simulink model "main2_2023b"  (R2023b)
settings: Solver=ode15s  StartTime=0.0  StopTime=15  MaxStep=1e-4  RelTol=1e-3
InitFcn:
  | parametros
values from neighbouring files (symbols this model uses):
  alpha_cu = 3.9 *10^-3    (= 0.0039)    [parametros.m]
  b_l = 0.1    [parametros.m]
  b_m = 1.5 * 10^-5    (= 1.5e-05)    [parametros.m]
  C_ts = 0.818    [parametros.m]
  J_l = (m*l_cm^2 + J_cm) + (m_l * l_l^2)    (= 0.0833)    [parametros.m]
  J_m = 1.4 * 10^-5    (= 1.4e-05)    [parametros.m]
  K_e_omega = 3*3200^2    (= 30720000)    [parametros.m]
  K_e_theta = 9600    [parametros.m]
  k_l = m * g * l_cm + m_l * g * l_l    (= 2.4516625)    [parametros.m]
  L_d = 6.6 * 10^-3    (= 0.0066)    [parametros.m]
  L_ls = 0.8 * 10^-3    (= 0.0008)    [parametros.m]
  L_q = 5.8 * 10^-3    (= 0.0058)    [parametros.m]
  lambda_m = 0.016    [parametros.m]
  P_p = 3    [parametros.m]
  r = 120    [parametros.m]
  R_s_40 = 1.02    [parametros.m]
  R_ts_amb = 146.7    [parametros.m]
  Temp_s_ref = 40    [parametros.m]
libraries: simulink x6
(part 2 of 2)

== system main2_2023b/5.2.1 ids = 3/Sensores ==
  theta_m : Inport
  T_s : Inport  Port=2
  i_as : Inport  Port=3
  i_bs : Inport  Port=4
  i_cs : Inport  Port=5
  Gain{,1..4} (5 alike) : Gain
  theta_m_medida : Outport
  T_s_medida : Outport  Port=2
  i_as_medida : Outport  Port=3
  i_bs_medida : Outport  Port=4
  i_cs_medida : Outport  Port=5
  wires:
  theta_m/1 -> Gain/1
  T_s/1 -> Gain1/1
  i_as/1 -> Gain2/1
  Gain/1 -> theta_m_medida/1
  Gain1/1 -> T_s_medida/1
  Gain2/1 -> i_as_medida/1
  Gain3/1 -> i_bs_medida/1
  i_bs/1 -> Gain3/1
  i_cs/1 -> Gain4/1
  Gain4/1 -> i_cs_medida/1

== system main2_2023b/5.2.1 ids = 3/Setpoint ==
  q1* : Inport
  Derivative : Derivative
  Gain : Gain  Gain=r
  theta_m* : Outport
  omega_m* : Outport  Port=2
  wires:
  q1*/1 -> Gain/1
  Gain/1 -> Derivative/1, theta_m*/1
  Derivative/1 -> omega_m*/1

== system main2_2023b/5.2.1 ids = 3/Subsistema físico no lineal  ==
  T_l : Inport
  v_as : Inport  Port=2
  v_bs : Inport  Port=3
  v_cs : Inport  Port=4
  theta_r : Inport  Port=5
  Tº_amb : Inport  Port=6
  Subsistema electromagnético : Subsystem
  Subsistema mecánico completo : Subsystem
  Subsistema térmico : Subsystem
  TD_PARK : MATLAB Function  TreatAsAtomicUnit=on
  TI_PARK : MATLAB Function  TreatAsAtomicUnit=on
  theta_m : Outport
  T_s : Outport  Port=2
  i_as : Outport  Port=3
  i_bs : Outport  Port=4
  i_cs : Outport  Port=5
  omega_m : Outport  Port=6
  T_m : Outport  Port=7
  wires:
  theta_r/1 -> TI_PARK/4(theta_r), TD_PARK/4(theta_r)
  TI_PARK/2(fbs) -> i_bs/1
  v_cs/1 -> TD_PARK/3(fcs)
  v_as/1 -> TD_PARK/1(fas)
  TI_PARK/3(fcs) -> i_cs/1
  v_bs/1 -> TD_PARK/2(fbs)
  TI_PARK/1(fas) -> i_as/1
  TD_PARK/1(fqs) -> Subsistema electromagnético/1(v_qs^r)
  TD_PARK/2(fds) -> Subsistema electromagnético/2(v_ds^r)
  TD_PARK/3(f0s) -> Subsistema electromagnético/3(v_0s^r)
  Subsistema mecánico completo/2(omega_m(t)) -> Subsistema electromagnético/4(omega_m), omega_m/1
  Subsistema térmico/2(r_s) -> Subsistema electromagnético/5(r_s)
  Subsistema electromagnético/2(i_ds^r) -> Subsistema térmico/2(i_ds^r), TI_PARK/2(fds)
  Subsistema electromagnético/3(i_qs^r) -> Subsistema térmico/1(i_qs^r), TI_PARK/1(fqs)
  Subsistema electromagnético/1(i_0s^r) -> Subsistema térmico/3(i_0s^r), TI_PARK/3(f0s)
  Subsistema electromagnético/4(T_m) -> Subsistema mecánico completo/1(T_m), T_m/1
  T_l/1 -> Subsistema mecánico completo/2(T_l)
  Tº_amb/1 -> Subsistema térmico/4(Tº_amb)
  Subsistema térmico/1(T_s) -> T_s/1
  Subsistema mecánico completo/1(theta_m(t)) -> theta_m/1

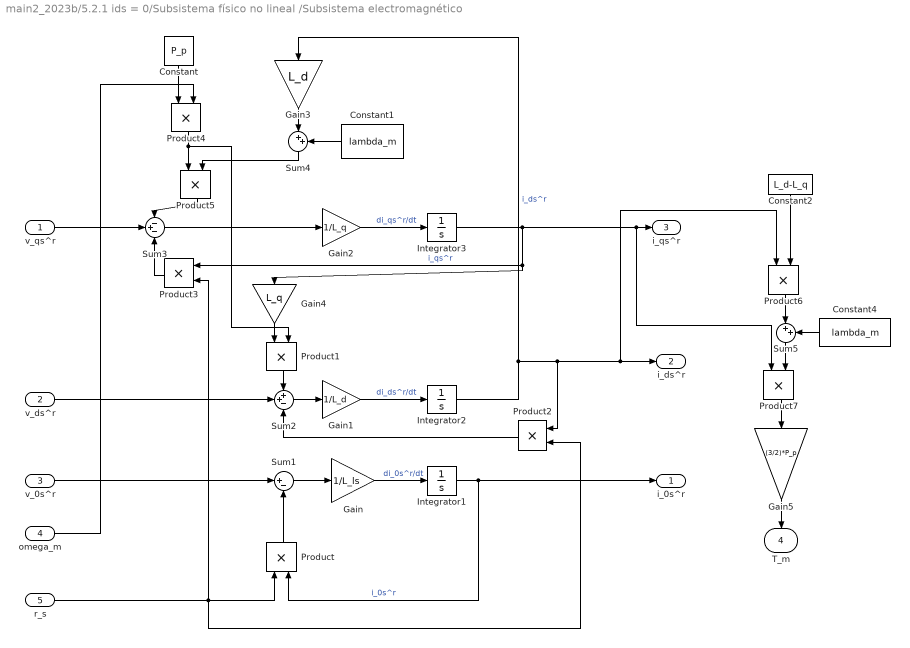
== system main2_2023b/5.2.1 ids = 0/Subsistema físico no lineal /Subsistema electromagnético ==
  v_qs^r : Inport
  v_ds^r : Inport  Port=2
  v_0s^r : Inport  Port=3
  omega_m : Inport  Port=4
  r_s : Inport  Port=5
  Constant : Constant  Value=P_p
  Constant1 : Constant  Value=lambda_m
  Constant2 : Constant  Value=L_d-L_q
  Constant4 : Constant  Value=lambda_m
  Gain : Gain  Gain=1/L_ls
  Gain1 : Gain  Gain=1/L_d
  Gain2 : Gain  Gain=1/L_q
  Gain3 : Gain  Gain=L_d
  Gain4 : Gain  Gain=L_q
  Gain5 : Gain  Gain=(3/2)*P_p
  Integrator1 : Integrator
  Integrator2 : Integrator
  Integrator3 : Integrator
  Product{,1..7} (8 alike) : Product
  Sum1 : Sum  Inputs=|+-
  Sum2 : Sum  Inputs=++-
  Sum3 : Sum  Inputs=-+-
  Sum4 : Sum  Inputs=|++
  Sum5 : Sum  Inputs=|++
  i_0s^r : Outport
  i_ds^r : Outport  Port=2
  i_qs^r : Outport  Port=3
  T_m : Outport  Port=4
  wires:
  Constant2/1 -> Product6/2
  Gain5/1 -> T_m/1
  Product5/1 -> Sum3/1
  Product2/1 -> Sum2/3
  Product6/1 -> Sum5/1
  Product1/1 -> Sum2/1
  Gain4/1 -> Product1/1
  Constant4/1 -> Sum5/2
  Sum3/1 -> Gain2/1
  Constant1/1 -> Sum4/2
  Integrator1/1 -> i_0s^r/1, Product/2  "i_0s^r"
  v_ds^r/1 -> Sum2/2
  Product4/1 -> Product1/2, Product5/1
  Sum5/1 -> Product7/2
  Product7/1 -> Gain5/1
  Integrator2/1 -> Gain3/1, Product2/1, Product6/1, i_ds^r/1  "i_ds^r"
  Sum4/1 -> Product5/2
  Product/1 -> Sum1/2
  Integrator3/1 -> Product3/1, Gain4/1, Product7/1, i_qs^r/1  "i_qs^r"
  Product3/1 -> Sum3/3
  Gain/1 -> Integrator1/1  "di_0s^r/dt"
  Gain3/1 -> Sum4/1
  omega_m/1 -> Product4/2
  Constant/1 -> Product4/1
  Sum1/1 -> Gain/1
  r_s/1 -> Product3/2, Product2/2, Product/1
  v_qs^r/1 -> Sum3/2
  Gain2/1 -> Integrator3/1  "di_qs^r/dt"
  v_0s^r/1 -> Sum1/1
  Gain1/1 -> Integrator2/1  "di_ds^r/dt"
  Sum2/1 -> Gain1/1

== system main2_2023b/5.2.1 ids = 0/Subsistema físico no lineal /Subsistema mecánico completo ==
  T_m : Inport
  T_l : Inport  Port=2
  Gain : Gain  Gain=b_m +( b_l / (r^2))
  Gain1 : Gain  Gain=1/r
  Gain2 : Gain  Gain=1/(J_m + J_l / (r^2))
  Sum : Sum  Inputs=-+-
  omega_m(0) = 0 : Integrator
  theta_m(0) = 0 : Integrator
  theta_m(t) : Outport
  omega_m(t) : Outport  Port=2
  wires:
  Gain2/1 -> omega_m(0) = 0/1  "domega_m(t)/dt"
  Gain1/1 -> Sum/1
  theta_m(0) = 0/1 -> theta_m(t)/1  "theta_m(t)"
  omega_m(0) = 0/1 -> omega_m(t)/1, Gain/1, theta_m(0) = 0/1  "omega_m(t)"
  Sum/1 -> Gain2/1
  Gain/1 -> Sum/3
  T_l/1 -> Gain1/1
  T_m/1 -> Sum/2

== system main2_2023b/5.2.1 ids = 0/Subsistema físico no lineal /Subsistema térmico ==
  i_qs^r : Inport
  i_ds^r : Inport  Port=2
  i_0s^r : Inport  Port=3
  Tº_amb : Inport  Port=4
  CI = 40ºC : Integrator  InitialCondition=40
  Constant : Constant
  Gain : Gain  Gain=1/C_ts
  Gain1 : Gain  Gain=2
  Gain2 : Gain  Gain=3/2
  Gain3 : Gain  Gain=1/R_ts_amb
  Gain4 : Gain  Gain=alpha_cu
  Gain5 : Gain  Gain=R_s_40
  Product : Product
  Square : Math  Operator=square
  Square1 : Math  Operator=square
  Square2 : Math  Operator=square
  Sum : Sum  Inputs=+++
  Sum1 : Sum  Inputs=|+-
  Sum2 : Sum  Inputs=|-+
  Sum3 : Sum  Inputs=|++
  T_s : Outport
  r_s : Outport  Port=2
  wires:
  CI = 40ºC/1 -> Sum2/2, T_s/1
  Gain/1 -> CI = 40ºC/1
  Sum1/1 -> Gain/1
  i_qs^r/1 -> Square/1
  i_ds^r/1 -> Square1/1
  i_0s^r/1 -> Square2/1
  Square2/1 -> Gain1/1
  Square/1 -> Sum/1
  Square1/1 -> Sum/2
  Gain1/1 -> Sum/3
  Gain5/1 -> r_s/1, Gain2/1
  Gain2/1 -> Product/2
  Sum/1 -> Product/1
  Product/1 -> Sum1/1
  Tº_amb/1 -> Sum2/1
  Sum2/1 -> Gain4/1, Gain3/1
  Gain3/1 -> Sum1/2
  Gain4/1 -> Sum3/1
  Constant/1 -> Sum3/2
  Sum3/1 -> Gain5/1

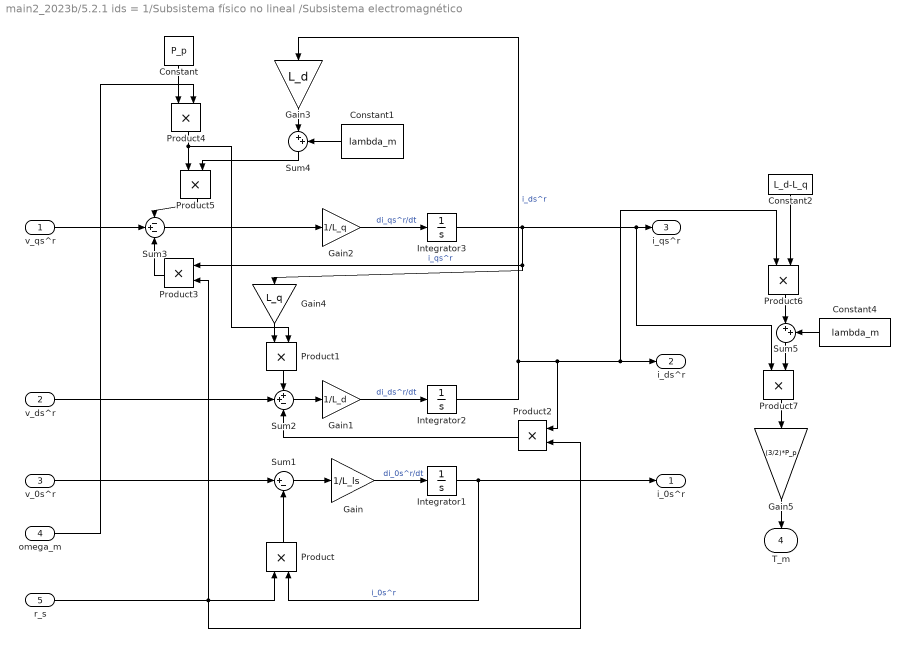
== system main2_2023b/5.2.1 ids = 1/Subsistema físico no lineal /Subsistema electromagnético ==
  v_qs^r : Inport
  v_ds^r : Inport  Port=2
  v_0s^r : Inport  Port=3
  omega_m : Inport  Port=4
  r_s : Inport  Port=5
  Constant : Constant  Value=P_p
  Constant1 : Constant  Value=lambda_m
  Constant2 : Constant  Value=L_d-L_q
  Constant4 : Constant  Value=lambda_m
  Gain : Gain  Gain=1/L_ls
  Gain1 : Gain  Gain=1/L_d
  Gain2 : Gain  Gain=1/L_q
  Gain3 : Gain  Gain=L_d
  Gain4 : Gain  Gain=L_q
  Gain5 : Gain  Gain=(3/2)*P_p
  Integrator1 : Integrator
  Integrator2 : Integrator
  Integrator3 : Integrator
  Product{,1..7} (8 alike) : Product
  Sum1 : Sum  Inputs=|+-
  Sum2 : Sum  Inputs=++-
  Sum3 : Sum  Inputs=-+-
  Sum4 : Sum  Inputs=|++
  Sum5 : Sum  Inputs=|++
  i_0s^r : Outport
  i_ds^r : Outport  Port=2
  i_qs^r : Outport  Port=3
  T_m : Outport  Port=4
  wires:
  Constant2/1 -> Product6/2
  Gain5/1 -> T_m/1
  Product5/1 -> Sum3/1
  Product2/1 -> Sum2/3
  Product6/1 -> Sum5/1
  Product1/1 -> Sum2/1
  Gain4/1 -> Product1/1
  Constant4/1 -> Sum5/2
  Sum3/1 -> Gain2/1
  Constant1/1 -> Sum4/2
  Integrator1/1 -> i_0s^r/1, Product/2  "i_0s^r"
  v_ds^r/1 -> Sum2/2
  Product4/1 -> Product1/2, Product5/1
  Sum5/1 -> Product7/2
  Product7/1 -> Gain5/1
  Integrator2/1 -> Gain3/1, Product2/1, Product6/1, i_ds^r/1  "i_ds^r"
  Sum4/1 -> Product5/2
  Product/1 -> Sum1/2
  Integrator3/1 -> Product3/1, Gain4/1, Product7/1, i_qs^r/1  "i_qs^r"
  Product3/1 -> Sum3/3
  Gain/1 -> Integrator1/1  "di_0s^r/dt"
  Gain3/1 -> Sum4/1
  omega_m/1 -> Product4/2
  Constant/1 -> Product4/1
  Sum1/1 -> Gain/1
  r_s/1 -> Product3/2, Product2/2, Product/1
  v_qs^r/1 -> Sum3/2
  Gain2/1 -> Integrator3/1  "di_qs^r/dt"
  v_0s^r/1 -> Sum1/1
  Gain1/1 -> Integrator2/1  "di_ds^r/dt"
  Sum2/1 -> Gain1/1

== system main2_2023b/5.2.1 ids = 1/Subsistema físico no lineal /Subsistema mecánico completo ==
  T_m : Inport
  T_l : Inport  Port=2
  Gain : Gain  Gain=b_m +( b_l / (r^2))
  Gain1 : Gain  Gain=1/r
  Gain2 : Gain  Gain=1/(J_m + J_l / (r^2))
  Sum : Sum  Inputs=-+-
  omega_m(0) = 0 : Integrator
  theta_m(0) = 0 : Integrator
  theta_m(t) : Outport
  omega_m(t) : Outport  Port=2
  wires:
  Gain2/1 -> omega_m(0) = 0/1  "domega_m(t)/dt"
  Gain1/1 -> Sum/1
  theta_m(0) = 0/1 -> theta_m(t)/1  "theta_m(t)"
  omega_m(0) = 0/1 -> omega_m(t)/1, Gain/1, theta_m(0) = 0/1  "omega_m(t)"
  Sum/1 -> Gain2/1
  Gain/1 -> Sum/3
  T_l/1 -> Gain1/1
  T_m/1 -> Sum/2

== system main2_2023b/5.2.1 ids = 1/Subsistema físico no lineal /Subsistema térmico ==
  i_qs^r : Inport
  i_ds^r : Inport  Port=2
  i_0s^r : Inport  Port=3
  Tº_amb : Inport  Port=4
  CI = 40ºC : Integrator  InitialCondition=40
  Constant : Constant
  Gain : Gain  Gain=1/C_ts
  Gain1 : Gain  Gain=2
  Gain2 : Gain  Gain=3/2
  Gain3 : Gain  Gain=1/R_ts_amb
  Gain4 : Gain  Gain=alpha_cu
  Gain5 : Gain  Gain=R_s_40
  Product : Product
  Square : Math  Operator=square
  Square1 : Math  Operator=square
  Square2 : Math  Operator=square
  Sum : Sum  Inputs=+++
  Sum1 : Sum  Inputs=|+-
  Sum2 : Sum  Inputs=|-+
  Sum3 : Sum  Inputs=|++
  T_s : Outport
  r_s : Outport  Port=2
  wires:
  CI = 40ºC/1 -> Sum2/2, T_s/1
  Gain/1 -> CI = 40ºC/1
  Sum1/1 -> Gain/1
  i_qs^r/1 -> Square/1
  i_ds^r/1 -> Square1/1
  i_0s^r/1 -> Square2/1
  Square2/1 -> Gain1/1
  Square/1 -> Sum/1
  Square1/1 -> Sum/2
  Gain1/1 -> Sum/3
  Gain5/1 -> r_s/1, Gain2/1
  Gain2/1 -> Product/2
  Sum/1 -> Product/1
  Product/1 -> Sum1/1
  Tº_amb/1 -> Sum2/1
  Sum2/1 -> Gain4/1, Gain3/1
  Gain3/1 -> Sum1/2
  Gain4/1 -> Sum3/1
  Constant/1 -> Sum3/2
  Sum3/1 -> Gain5/1

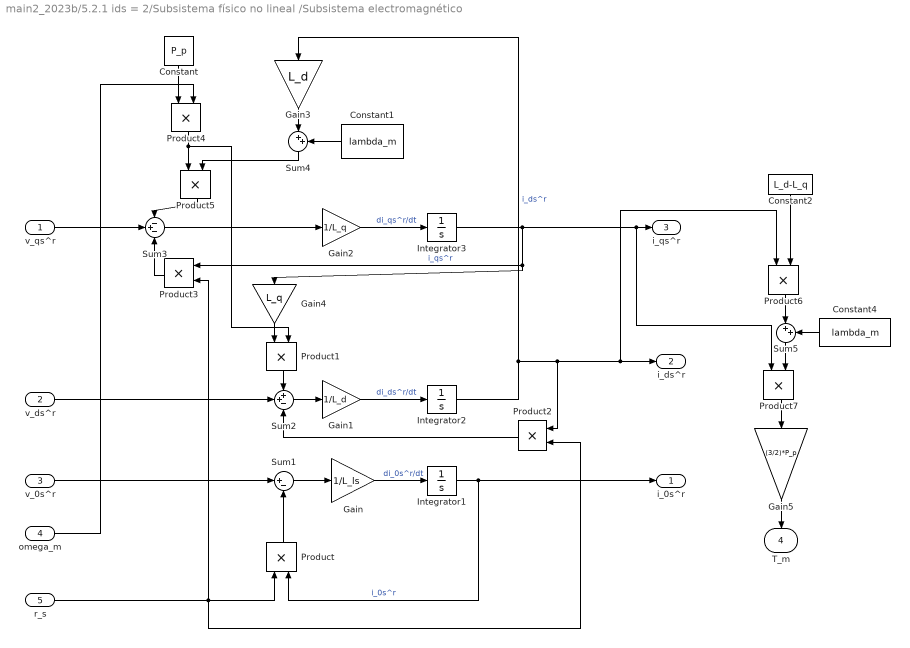
== system main2_2023b/5.2.1 ids = 2/Subsistema físico no lineal /Subsistema electromagnético ==
  v_qs^r : Inport
  v_ds^r : Inport  Port=2
  v_0s^r : Inport  Port=3
  omega_m : Inport  Port=4
  r_s : Inport  Port=5
  Constant : Constant  Value=P_p
  Constant1 : Constant  Value=lambda_m
  Constant2 : Constant  Value=L_d-L_q
  Constant4 : Constant  Value=lambda_m
  Gain : Gain  Gain=1/L_ls
  Gain1 : Gain  Gain=1/L_d
  Gain2 : Gain  Gain=1/L_q
  Gain3 : Gain  Gain=L_d
  Gain4 : Gain  Gain=L_q
  Gain5 : Gain  Gain=(3/2)*P_p
  Integrator1 : Integrator
  Integrator2 : Integrator
  Integrator3 : Integrator
  Product{,1..7} (8 alike) : Product
  Sum1 : Sum  Inputs=|+-
  Sum2 : Sum  Inputs=++-
  Sum3 : Sum  Inputs=-+-
  Sum4 : Sum  Inputs=|++
  Sum5 : Sum  Inputs=|++
  i_0s^r : Outport
  i_ds^r : Outport  Port=2
  i_qs^r : Outport  Port=3
  T_m : Outport  Port=4
  wires:
  Constant2/1 -> Product6/2
  Gain5/1 -> T_m/1
  Product5/1 -> Sum3/1
  Product2/1 -> Sum2/3
  Product6/1 -> Sum5/1
  Product1/1 -> Sum2/1
  Gain4/1 -> Product1/1
  Constant4/1 -> Sum5/2
  Sum3/1 -> Gain2/1
  Constant1/1 -> Sum4/2
  Integrator1/1 -> i_0s^r/1, Product/2  "i_0s^r"
  v_ds^r/1 -> Sum2/2
  Product4/1 -> Product1/2, Product5/1
  Sum5/1 -> Product7/2
  Product7/1 -> Gain5/1
  Integrator2/1 -> Gain3/1, Product2/1, Product6/1, i_ds^r/1  "i_ds^r"
  Sum4/1 -> Product5/2
  Product/1 -> Sum1/2
  Integrator3/1 -> Product3/1, Gain4/1, Product7/1, i_qs^r/1  "i_qs^r"
  Product3/1 -> Sum3/3
  Gain/1 -> Integrator1/1  "di_0s^r/dt"
  Gain3/1 -> Sum4/1
  omega_m/1 -> Product4/2
  Constant/1 -> Product4/1
  Sum1/1 -> Gain/1
  r_s/1 -> Product3/2, Product2/2, Product/1
  v_qs^r/1 -> Sum3/2
  Gain2/1 -> Integrator3/1  "di_qs^r/dt"
  v_0s^r/1 -> Sum1/1
  Gain1/1 -> Integrator2/1  "di_ds^r/dt"
  Sum2/1 -> Gain1/1

== system main2_2023b/5.2.1 ids = 2/Subsistema físico no lineal /Subsistema mecánico completo ==
  T_m : Inport
  T_l : Inport  Port=2
  Gain : Gain  Gain=b_m +( b_l / (r^2))
  Gain1 : Gain  Gain=1/r
  Gain2 : Gain  Gain=1/(J_m + J_l / (r^2))
  Sum : Sum  Inputs=-+-
  omega_m(0) = 0 : Integrator
  theta_m(0) = 0 : Integrator
  theta_m(t) : Outport
  omega_m(t) : Outport  Port=2
  wires:
  Gain2/1 -> omega_m(0) = 0/1  "domega_m(t)/dt"
  Gain1/1 -> Sum/1
  theta_m(0) = 0/1 -> theta_m(t)/1  "theta_m(t)"
  omega_m(0) = 0/1 -> omega_m(t)/1, Gain/1, theta_m(0) = 0/1  "omega_m(t)"
  Sum/1 -> Gain2/1
  Gain/1 -> Sum/3
  T_l/1 -> Gain1/1
  T_m/1 -> Sum/2

== system main2_2023b/5.2.1 ids = 2/Subsistema físico no lineal /Subsistema térmico ==
  i_qs^r : Inport
  i_ds^r : Inport  Port=2
  i_0s^r : Inport  Port=3
  Tº_amb : Inport  Port=4
  CI = 40ºC : Integrator  InitialCondition=40
  Constant : Constant
  Gain : Gain  Gain=1/C_ts
  Gain1 : Gain  Gain=2
  Gain2 : Gain  Gain=3/2
  Gain3 : Gain  Gain=1/R_ts_amb
  Gain4 : Gain  Gain=alpha_cu
  Gain5 : Gain  Gain=R_s_40
  Product : Product
  Square : Math  Operator=square
  Square1 : Math  Operator=square
  Square2 : Math  Operator=square
  Sum : Sum  Inputs=+++
  Sum1 : Sum  Inputs=|+-
  Sum2 : Sum  Inputs=|-+
  Sum3 : Sum  Inputs=|++
  T_s : Outport
  r_s : Outport  Port=2
  wires:
  CI = 40ºC/1 -> Sum2/2, T_s/1
  Gain/1 -> CI = 40ºC/1
  Sum1/1 -> Gain/1
  i_qs^r/1 -> Square/1
  i_ds^r/1 -> Square1/1
  i_0s^r/1 -> Square2/1
  Square2/1 -> Gain1/1
  Square/1 -> Sum/1
  Square1/1 -> Sum/2
  Gain1/1 -> Sum/3
  Gain5/1 -> r_s/1, Gain2/1
  Gain2/1 -> Product/2
  Sum/1 -> Product/1
  Product/1 -> Sum1/1
  Tº_amb/1 -> Sum2/1
  Sum2/1 -> Gain4/1, Gain3/1
  Gain3/1 -> Sum1/2
  Gain4/1 -> Sum3/1
  Constant/1 -> Sum3/2
  Sum3/1 -> Gain5/1

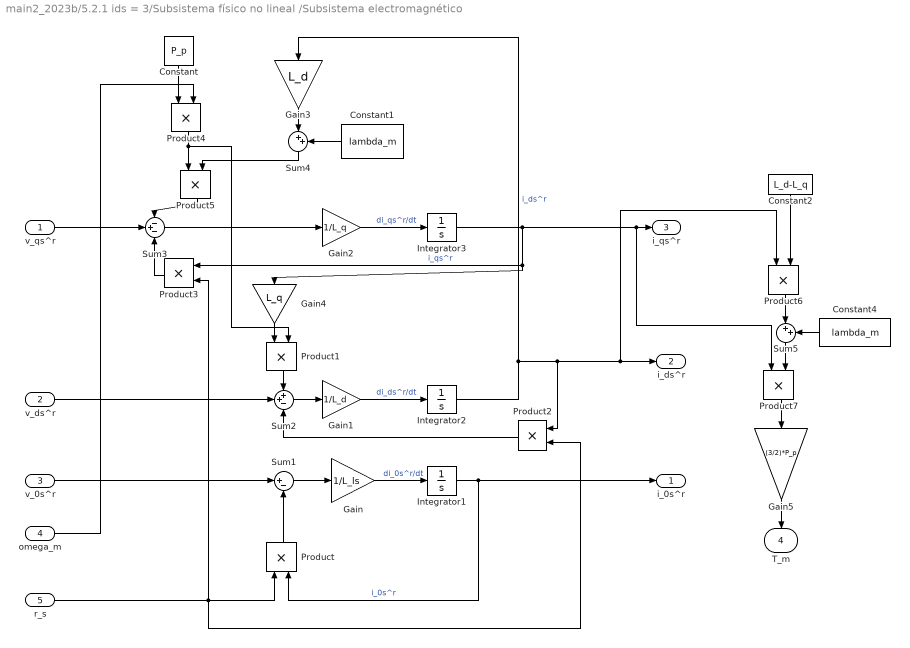
== system main2_2023b/5.2.1 ids = 3/Subsistema físico no lineal /Subsistema electromagnético ==
  v_qs^r : Inport
  v_ds^r : Inport  Port=2
  v_0s^r : Inport  Port=3
  omega_m : Inport  Port=4
  r_s : Inport  Port=5
  Constant : Constant  Value=P_p
  Constant1 : Constant  Value=lambda_m
  Constant2 : Constant  Value=L_d-L_q
  Constant4 : Constant  Value=lambda_m
  Gain : Gain  Gain=1/L_ls
  Gain1 : Gain  Gain=1/L_d
  Gain2 : Gain  Gain=1/L_q
  Gain3 : Gain  Gain=L_d
  Gain4 : Gain  Gain=L_q
  Gain5 : Gain  Gain=(3/2)*P_p
  Integrator1 : Integrator
  Integrator2 : Integrator
  Integrator3 : Integrator
  Product{,1..7} (8 alike) : Product
  Sum1 : Sum  Inputs=|+-
  Sum2 : Sum  Inputs=++-
  Sum3 : Sum  Inputs=-+-
  Sum4 : Sum  Inputs=|++
  Sum5 : Sum  Inputs=|++
  i_0s^r : Outport
  i_ds^r : Outport  Port=2
  i_qs^r : Outport  Port=3
  T_m : Outport  Port=4
  wires:
  Constant2/1 -> Product6/2
  Gain5/1 -> T_m/1
  Product5/1 -> Sum3/1
  Product2/1 -> Sum2/3
  Product6/1 -> Sum5/1
  Product1/1 -> Sum2/1
  Gain4/1 -> Product1/1
  Constant4/1 -> Sum5/2
  Sum3/1 -> Gain2/1
  Constant1/1 -> Sum4/2
  Integrator1/1 -> i_0s^r/1, Product/2  "i_0s^r"
  v_ds^r/1 -> Sum2/2
  Product4/1 -> Product1/2, Product5/1
  Sum5/1 -> Product7/2
  Product7/1 -> Gain5/1
  Integrator2/1 -> Gain3/1, Product2/1, Product6/1, i_ds^r/1  "i_ds^r"
  Sum4/1 -> Product5/2
  Product/1 -> Sum1/2
  Integrator3/1 -> Product3/1, Gain4/1, Product7/1, i_qs^r/1  "i_qs^r"
  Product3/1 -> Sum3/3
  Gain/1 -> Integrator1/1  "di_0s^r/dt"
  Gain3/1 -> Sum4/1
  omega_m/1 -> Product4/2
  Constant/1 -> Product4/1
  Sum1/1 -> Gain/1
  r_s/1 -> Product3/2, Product2/2, Product/1
  v_qs^r/1 -> Sum3/2
  Gain2/1 -> Integrator3/1  "di_qs^r/dt"
  v_0s^r/1 -> Sum1/1
  Gain1/1 -> Integrator2/1  "di_ds^r/dt"
  Sum2/1 -> Gain1/1

== system main2_2023b/5.2.1 ids = 3/Subsistema físico no lineal /Subsistema mecánico completo ==
  T_m : Inport
  T_l : Inport  Port=2
  Gain : Gain  Gain=b_m +( b_l / (r^2))
  Gain1 : Gain  Gain=1/r
  Gain2 : Gain  Gain=1/(J_m + J_l / (r^2))
  Sum : Sum  Inputs=-+-
  omega_m(0) = 0 : Integrator
  theta_m(0) = 0 : Integrator
  theta_m(t) : Outport
  omega_m(t) : Outport  Port=2
  wires:
  Gain2/1 -> omega_m(0) = 0/1  "domega_m(t)/dt"
  Gain1/1 -> Sum/1
  theta_m(0) = 0/1 -> theta_m(t)/1  "theta_m(t)"
  omega_m(0) = 0/1 -> omega_m(t)/1, Gain/1, theta_m(0) = 0/1  "omega_m(t)"
  Sum/1 -> Gain2/1
  Gain/1 -> Sum/3
  T_l/1 -> Gain1/1
  T_m/1 -> Sum/2

== system main2_2023b/5.2.1 ids = 3/Subsistema físico no lineal /Subsistema térmico ==
  i_qs^r : Inport
  i_ds^r : Inport  Port=2
  i_0s^r : Inport  Port=3
  Tº_amb : Inport  Port=4
  CI = 40ºC : Integrator  InitialCondition=40
  Constant : Constant
  Gain : Gain  Gain=1/C_ts
  Gain1 : Gain  Gain=2
  Gain2 : Gain  Gain=3/2
  Gain3 : Gain  Gain=1/R_ts_amb
  Gain4 : Gain  Gain=alpha_cu
  Gain5 : Gain  Gain=R_s_40
  Product : Product
  Square : Math  Operator=square
  Square1 : Math  Operator=square
  Square2 : Math  Operator=square
  Sum : Sum  Inputs=+++
  Sum1 : Sum  Inputs=|+-
  Sum2 : Sum  Inputs=|-+
  Sum3 : Sum  Inputs=|++
  T_s : Outport
  r_s : Outport  Port=2
  wires:
  CI = 40ºC/1 -> Sum2/2, T_s/1
  Gain/1 -> CI = 40ºC/1
  Sum1/1 -> Gain/1
  i_qs^r/1 -> Square/1
  i_ds^r/1 -> Square1/1
  i_0s^r/1 -> Square2/1
  Square2/1 -> Gain1/1
  Square/1 -> Sum/1
  Square1/1 -> Sum/2
  Gain1/1 -> Sum/3
  Gain5/1 -> r_s/1, Gain2/1
  Gain2/1 -> Product/2
  Sum/1 -> Product/1
  Product/1 -> Sum1/1
  Tº_amb/1 -> Sum2/1
  Sum2/1 -> Gain4/1, Gain3/1
  Gain3/1 -> Sum1/2
  Gain4/1 -> Sum3/1
  Constant/1 -> Sum3/2
  Sum3/1 -> Gain5/1

== matlab function main2_2023b/5.2.1 ids = 3/TD_PARK ==
  data: fas input; fqs output; fbs input; fcs input; theta_r input; fds output; f0s output
function [fqs, fds, f0s] = TD_PARK(fas, fbs, fcs, theta_r)

    fabcs = [fas; fbs; fcs];

    Ks = 2/3*[cos(theta_r) cos(theta_r - 2*pi/3) cos(theta_r + 2*pi/3)
          sin(theta_r) sin(theta_r - 2*pi/3) sin(theta_r + 2*pi/3) 
          1/2          1/2                   1/2];

    fqd0s = Ks * fabcs;

    fqs = fqd0s(1);
    fds = fqd0s(2);
    f0s = fqd0s(3);

end

== matlab function main2_2023b/5.2.1 ids = 0/Subsistema físico no lineal /TD_PARK ==
  data: fas input; fqs output; fbs input; fcs input; theta_r input; fds output; f0s output
function [fqs, fds, f0s] = TD_PARK(fas, fbs, fcs, theta_r)

    fabcs = [fas; fbs; fcs];

    Ks = 2/3*[cos(theta_r) cos(theta_r - 2*pi/3) cos(theta_r + 2*pi/3)
          sin(theta_r) sin(theta_r - 2*pi/3) sin(theta_r + 2*pi/3) 
          1/2          1/2                   1/2];

    fqd0s = Ks * fabcs;

    fqs = fqd0s(1);
    fds = fqd0s(2);
    f0s = fqd0s(3);

end

== matlab function main2_2023b/5.2.1 ids = 3/TI_PARK1 ==
  data: fqs input; fas output; fds input; f0s input; theta_r input; fbs output; fcs output
function [fas, fbs, fcs] = TI_PARK(fqs, fds, f0s , theta_r)

    fqd0s = [fqs; fds; f0s];

    Ks = [cos(theta_r)         sin(theta_r)             1
          cos(theta_r - 2*pi/3) sin(theta_r - 2*pi/3)    1
          cos(theta_r + 2*pi/3) sin(theta_r + 2*pi/3)    1];

    fabcs = Ks * fqd0s;

    fas = fabcs(1);
    fbs = fabcs(2);
    fcs = fabcs(3);

end

== matlab function main2_2023b/5.2.1 ids = 1/Subsistema físico no lineal /TD_PARK ==
  data: fas input; fqs output; fbs input; fcs input; theta_r input; fds output; f0s output
function [fqs, fds, f0s] = TD_PARK(fas, fbs, fcs, theta_r)

    fabcs = [fas; fbs; fcs];

    Ks = 2/3*[cos(theta_r) cos(theta_r - 2*pi/3) cos(theta_r + 2*pi/3)
          sin(theta_r) sin(theta_r - 2*pi/3) sin(theta_r + 2*pi/3) 
          1/2          1/2                   1/2];

    fqd0s = Ks * fabcs;

    fqs = fqd0s(1);
    fds = fqd0s(2);
    f0s = fqd0s(3);

end

== matlab function main2_2023b/5.2.1 ids = 1/Subsistema físico no lineal /TI_PARK ==
  data: fqs input; fas output; fds input; f0s input; theta_r input; fbs output; fcs output
function [fas, fbs, fcs] = TI_PARK(fqs, fds, f0s , theta_r)

    fqd0s = [fqs; fds; f0s];

    Ks = [cos(theta_r)         sin(theta_r)             1
          cos(theta_r - 2*pi/3) sin(theta_r - 2*pi/3)    1
          cos(theta_r + 2*pi/3) sin(theta_r + 2*pi/3)    1];

    fabcs = Ks * fqd0s;

    fas = fabcs(1);
    fbs = fabcs(2);
    fcs = fabcs(3);

end

== matlab function main2_2023b/5.2.1 ids = 0/TI_PARK1 ==
  data: fqs input; fas output; fds input; f0s input; theta_r input; fbs output; fcs output
function [fas, fbs, fcs] = TI_PARK(fqs, fds, f0s , theta_r)

    fqd0s = [fqs; fds; f0s];

    Ks = [cos(theta_r)         sin(theta_r)             1
          cos(theta_r - 2*pi/3) sin(theta_r - 2*pi/3)    1
          cos(theta_r + 2*pi/3) sin(theta_r + 2*pi/3)    1];

    fabcs = Ks * fqd0s;

    fas = fabcs(1);
    fbs = fabcs(2);
    fcs = fabcs(3);

end

== matlab function main2_2023b/5.2.1 ids = 0/TD_PARK ==
  data: fas input; fqs output; fbs input; fcs input; theta_r input; fds output; f0s output
function [fqs, fds, f0s] = TD_PARK(fas, fbs, fcs, theta_r)

    fabcs = [fas; fbs; fcs];

    Ks = 2/3*[cos(theta_r) cos(theta_r - 2*pi/3) cos(theta_r + 2*pi/3)
          sin(theta_r) sin(theta_r - 2*pi/3) sin(theta_r + 2*pi/3) 
          1/2          1/2                   1/2];

    fqd0s = Ks * fabcs;

    fqs = fqd0s(1);
    fds = fqd0s(2);
    f0s = fqd0s(3);

end

== matlab function main2_2023b/5.2.1 ids = 1/TD_PARK ==
  data: fas input; fqs output; fbs input; fcs input; theta_r input; fds output; f0s output
function [fqs, fds, f0s] = TD_PARK(fas, fbs, fcs, theta_r)

    fabcs = [fas; fbs; fcs];

    Ks = 2/3*[cos(theta_r) cos(theta_r - 2*pi/3) cos(theta_r + 2*pi/3)
          sin(theta_r) sin(theta_r - 2*pi/3) sin(theta_r + 2*pi/3) 
          1/2          1/2                   1/2];

    fqd0s = Ks * fabcs;

    fqs = fqd0s(1);
    fds = fqd0s(2);
    f0s = fqd0s(3);

end

== matlab function main2_2023b/5.2.1 ids = 1/TI_PARK1 ==
  data: fqs input; fas output; fds input; f0s input; theta_r input; fbs output; fcs output
function [fas, fbs, fcs] = TI_PARK(fqs, fds, f0s , theta_r)

    fqd0s = [fqs; fds; f0s];

    Ks = [cos(theta_r)         sin(theta_r)             1
          cos(theta_r - 2*pi/3) sin(theta_r - 2*pi/3)    1
          cos(theta_r + 2*pi/3) sin(theta_r + 2*pi/3)    1];

    fabcs = Ks * fqd0s;

    fas = fabcs(1);
    fbs = fabcs(2);
    fcs = fabcs(3);

end

== matlab function main2_2023b/5.2.1 ids = 0/Subsistema físico no lineal /TI_PARK ==
  data: fqs input; fas output; fds input; f0s input; theta_r input; fbs output; fcs output
function [fas, fbs, fcs] = TI_PARK(fqs, fds, f0s , theta_r)

    fqd0s = [fqs; fds; f0s];

    Ks = [cos(theta_r)         sin(theta_r)             1
          cos(theta_r - 2*pi/3) sin(theta_r - 2*pi/3)    1
          cos(theta_r + 2*pi/3) sin(theta_r + 2*pi/3)    1];

    fabcs = Ks * fqd0s;

    fas = fabcs(1);
    fbs = fabcs(2);
    fcs = fabcs(3);

end

== matlab function main2_2023b/5.2.1 ids = 2/Subsistema físico no lineal /TD_PARK ==
  data: fas input; fqs output; fbs input; fcs input; theta_r input; fds output; f0s output
function [fqs, fds, f0s] = TD_PARK(fas, fbs, fcs, theta_r)

    fabcs = [fas; fbs; fcs];

    Ks = 2/3*[cos(theta_r) cos(theta_r - 2*pi/3) cos(theta_r + 2*pi/3)
          sin(theta_r) sin(theta_r - 2*pi/3) sin(theta_r + 2*pi/3) 
          1/2          1/2                   1/2];

    fqd0s = Ks * fabcs;

    fqs = fqd0s(1);
    fds = fqd0s(2);
    f0s = fqd0s(3);

end

== matlab function main2_2023b/5.2.1 ids = 2/Subsistema físico no lineal /TI_PARK ==
  data: fqs input; fas output; fds input; f0s input; theta_r input; fbs output; fcs output
function [fas, fbs, fcs] = TI_PARK(fqs, fds, f0s , theta_r)

    fqd0s = [fqs; fds; f0s];

    Ks = [cos(theta_r)         sin(theta_r)             1
          cos(theta_r - 2*pi/3) sin(theta_r - 2*pi/3)    1
          cos(theta_r + 2*pi/3) sin(theta_r + 2*pi/3)    1];

    fabcs = Ks * fqd0s;

    fas = fabcs(1);
    fbs = fabcs(2);
    fcs = fabcs(3);

end

== matlab function main2_2023b/5.2.1 ids = 2/TD_PARK ==
  data: fas input; fqs output; fbs input; fcs input; theta_r input; fds output; f0s output
function [fqs, fds, f0s] = TD_PARK(fas, fbs, fcs, theta_r)

    fabcs = [fas; fbs; fcs];

    Ks = 2/3*[cos(theta_r) cos(theta_r - 2*pi/3) cos(theta_r + 2*pi/3)
          sin(theta_r) sin(theta_r - 2*pi/3) sin(theta_r + 2*pi/3) 
          1/2          1/2                   1/2];

    fqd0s = Ks * fabcs;

    fqs = fqd0s(1);
    fds = fqd0s(2);
    f0s = fqd0s(3);

end

== matlab function main2_2023b/5.2.1 ids = 2/TI_PARK1 ==
  data: fqs input; fas output; fds input; f0s input; theta_r input; fbs output; fcs output
function [fas, fbs, fcs] = TI_PARK(fqs, fds, f0s , theta_r)

    fqd0s = [fqs; fds; f0s];

    Ks = [cos(theta_r)         sin(theta_r)             1
          cos(theta_r - 2*pi/3) sin(theta_r - 2*pi/3)    1
          cos(theta_r + 2*pi/3) sin(theta_r + 2*pi/3)    1];

    fabcs = Ks * fqd0s;

    fas = fabcs(1);
    fbs = fabcs(2);
    fcs = fabcs(3);

end

== matlab function main2_2023b/5.2.1 ids = 3/Subsistema físico no lineal /TD_PARK ==
  data: fas input; fqs output; fbs input; fcs input; theta_r input; fds output; f0s output
function [fqs, fds, f0s] = TD_PARK(fas, fbs, fcs, theta_r)

    fabcs = [fas; fbs; fcs];

    Ks = 2/3*[cos(theta_r) cos(theta_r - 2*pi/3) cos(theta_r + 2*pi/3)
          sin(theta_r) sin(theta_r - 2*pi/3) sin(theta_r + 2*pi/3) 
          1/2          1/2                   1/2];

    fqd0s = Ks * fabcs;

    fqs = fqd0s(1);
    fds = fqd0s(2);
    f0s = fqd0s(3);

end

== matlab function main2_2023b/5.2.1 ids = 3/Subsistema físico no lineal /TI_PARK ==
  data: fqs input; fas output; fds input; f0s input; theta_r input; fbs output; fcs output
function [fas, fbs, fcs] = TI_PARK(fqs, fds, f0s , theta_r)

    fqd0s = [fqs; fds; f0s];

    Ks = [cos(theta_r)         sin(theta_r)             1
          cos(theta_r - 2*pi/3) sin(theta_r - 2*pi/3)    1
          cos(theta_r + 2*pi/3) sin(theta_r + 2*pi/3)    1];

    fabcs = Ks * fqd0s;

    fas = fabcs(1);
    fbs = fabcs(2);
    fcs = fabcs(3);

end
